simulink model "Simulink_30_09"  (R2020a)
settings: Solver=VariableStepAuto  StartTime=0.0  StopTime=75  RelTol=1e-3
values from neighbouring files (symbols this model uses):
  K_LQR = Ks(:,[1:2])    [Script_LQR.m]    (also in Workspace_21_09.mat = [0.405324117713 1.57304723801]; Workspace_23_09.mat = [0.405324117713 1.57304723801]; Workspace_30_09.mat = [7.00831546655 5.45122974139]; Workspace_30_09_1.mat = [0.406231829475 1.23772711101])
  K_REI = [Ks(:,1) Ks(:,2)]    [Retro_Alimentacion_Integral.m]    (also in Workspace_30_09.mat = [5.59001533188 7.18657171923]; Workspace_30_09_1.mat = [5.59001533188 7.18657171923])
  Kd_ms = 0.1649    [Workspace_30_09.mat]    (also in Workspace_30_09_1.mat)
  Ki_LQR = -Ks(:,[3])    [Script_LQR.m]    (also in Workspace_21_09.mat = 1; Workspace_23_09.mat = 1; Workspace_30_09.mat = 5.9160797831; Workspace_30_09_1.mat = 1.18321595662)
  Ki_ms = 0.6328    [Workspace_30_09.mat]    (also in Workspace_30_09_1.mat)
  Ki_REI = -Ks(:,3)    [Retro_Alimentacion_Integral.m]    (also in Workspace_30_09.mat = 10.5317472521; Workspace_30_09_1.mat = 10.5317472521)
  Kp_ms = -0.2794    [Workspace_30_09.mat]    (also in Workspace_30_09_1.mat)
libraries: cstblocks x6, simulink x3
settings Model: Creator=geral  LastModifiedBy=geral

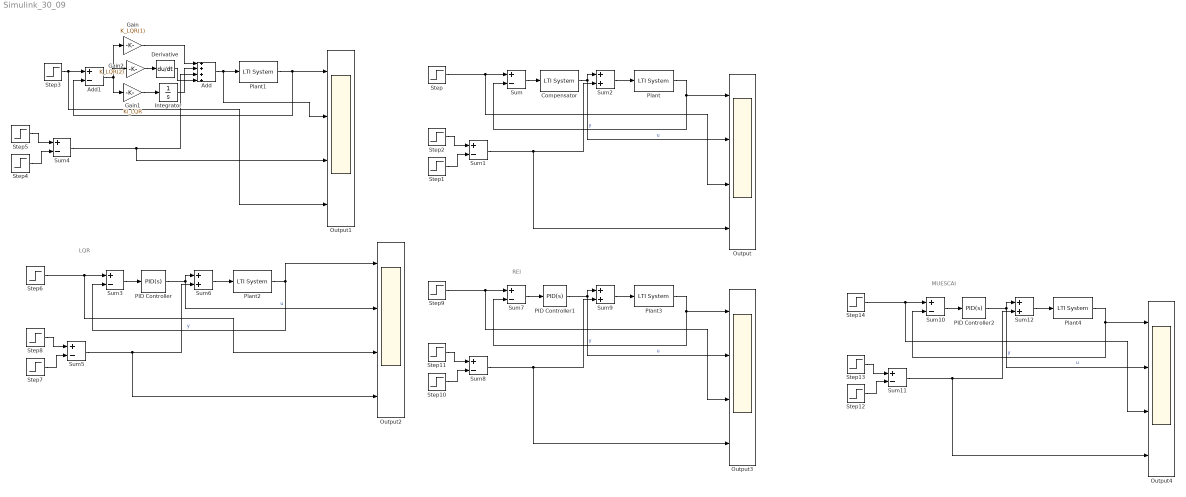
== system Simulink_30_09 ==
  note: REI
  note: LQR
  note: MUESCAI
  Add : Sum  Inputs=++++
  Add1 : Sum  Inputs=+-
  Compensator : cstblocks/LTI System  sys=C_IMC  IC=[]
  Derivative : Derivative
  Gain : Gain  Gain=K_LQR(1)
  Gain1 : Gain  Gain=Ki_LQR
  Gain2 : Gain  Gain=K_LQR(2)
  Integrator : Integrator
  Output{,1..4} (5 alike) : Scope  NumInputPorts=4
  PID Controller : simulink/Continuous/PID Controller  Controller=PID  Form=Parallel  TimeDomain=Continuous-time  UseExternalTs=off  SampleTime=-1  IntegratorMethod=Forward Euler  FilterMethod=Forward Euler  ControllerParametersSource=internal  P=K_LQR(1)  I=Ki_LQR  D=K_LQR(2)  UseFilter=on  N=15  TunerSelectOption=Transfer Function Based (PID Tuner App)  InitialConditionSource=internal  InitialConditionForIntegrator=0  InitialConditionForFilter=0  DifferentiatorICPrevScaledInput=0  ExternalReset=none  TrackingMode=off  Kt=1  LimitOutput=off  UpperSaturationLimit=inf  LowerSaturationLimit=-inf  LinearizeAsGain=on  AntiWindupMode=none  Kb=1  POutMin=[]  POutMax=[]  IOutMin=[]  IOutMax=[]  DOutMin=[]  DOutMax=[]  NOutMin=[]  NOutMax=[]  SumOutMin=[]  SumOutMax=[]  SaturationOutMin=[]  SaturationOutMax=[]  PParamMin=[]  PParamMax=[]  IParamMin=[]  IParamMax=[]  DParamMin=[]  DParamMax=[]  NParamMin=[]  NParamMax=[]  KbParamMin=[]  KbParamMax=[]  KtParamMin=[]  KtParamMax=[]  KbOutMin=[]  KbOutMax=[]  KtOutMin=[]  KtOutMax=[]  IntegratorOutMin=[]  IntegratorOutMax=[]  FilterOutMin=[]  FilterOutMax=[]  SumI1OutMin=[]  SumI1OutMax=[]  SumI2OutMin=[]  SumI2OutMax=[]  SumI3OutMin=[]  SumI3OutMax=[]  SumI4OutMin=[]  SumI4OutMax=[]  SumDOutMin=[]  SumDOutMax=[]  DifferentiatorOutMin=[]  DifferentiatorOutMax=[]  FilterDiffOutCoefMin=[]  FilterDiffOutCoefMax=[]  ReciprocalOutMin=[]  ReciprocalOutMax=[]  SumDenOutMin=[]  SumDenOutMax=[]  SumNumOutMin=[]  SumNumOutMax=[]  DivideOutMin=[]  DivideOutMax=[]  UdiffTsProdOutMin=[]  UdiffTsProdOutMax=[]  NTsProdOutMin=[]  NTsProdOutMax=[]  UintegralTsProdOutMin=[]  UintegralTsProdOutMax=[]  UngainTsProdOutMin=[]  UngainTsProdOutMax=[]  IntegratorContinuousStateAttributes=''  IntegratorStateMustResolveToSignalObject=off  IntegratorRTWStateStorageClass=Auto  FilterContinuousStateAttributes=''  FilterStateMustResolveToSignalObject=off  FilterRTWStateStorageClass=Auto  ParallelPVariant=InternalParameters  IdealPVariant=Disabled  IVariant=InternalParameters  DVariant=InternalParameters  IntegratorVariant=Continuous  SatVariant=Disabled  AWVariant=Passthrough  PCopyVariant=Disabled  TRVariant=Disabled  FdbkBlocksVariant=Forward  IdealPFdbkVariant=Disabled  SatFdbkVariant=Disabled  DerivativeFilterVariant=ContFilter  NVariant=InternalParameters  NCopyVariant=Disabled  FilterICVariant=InternalICsFilter  IntegratorICVariant=InternalICs  ExternalResetVariant=Disabled  TRSumVariant=Passthrough  SumFdbkVariant=Disabled  SumVariant=Sum_PID  TsampFilterVariant=InternalTs  TsampNgainVariant=Passthrough  TsampIntegralVariant=Passthrough
  PID Controller1 : simulink/Continuous/PID Controller  Controller=PID  Form=Parallel  TimeDomain=Continuous-time  UseExternalTs=off  SampleTime=-1  IntegratorMethod=Forward Euler  FilterMethod=Forward Euler  ControllerParametersSource=internal  P=K_REI(1)  I=Ki_REI  D=K_REI(2)  UseFilter=on  N=8.4  TunerSelectOption=Transfer Function Based (PID Tuner App)  InitialConditionSource=internal  InitialConditionForIntegrator=0  InitialConditionForFilter=0  DifferentiatorICPrevScaledInput=0  ExternalReset=none  TrackingMode=off  Kt=1  LimitOutput=off  UpperSaturationLimit=inf  LowerSaturationLimit=-inf  LinearizeAsGain=on  AntiWindupMode=none  Kb=1  POutMin=[]  POutMax=[]  IOutMin=[]  IOutMax=[]  DOutMin=[]  DOutMax=[]  NOutMin=[]  NOutMax=[]  SumOutMin=[]  SumOutMax=[]  SaturationOutMin=[]  SaturationOutMax=[]  PParamMin=[]  PParamMax=[]  IParamMin=[]  IParamMax=[]  DParamMin=[]  DParamMax=[]  NParamMin=[]  NParamMax=[]  KbParamMin=[]  KbParamMax=[]  KtParamMin=[]  KtParamMax=[]  KbOutMin=[]  KbOutMax=[]  KtOutMin=[]  KtOutMax=[]  IntegratorOutMin=[]  IntegratorOutMax=[]  FilterOutMin=[]  FilterOutMax=[]  SumI1OutMin=[]  SumI1OutMax=[]  SumI2OutMin=[]  SumI2OutMax=[]  SumI3OutMin=[]  SumI3OutMax=[]  SumI4OutMin=[]  SumI4OutMax=[]  SumDOutMin=[]  SumDOutMax=[]  DifferentiatorOutMin=[]  DifferentiatorOutMax=[]  FilterDiffOutCoefMin=[]  FilterDiffOutCoefMax=[]  ReciprocalOutMin=[]  ReciprocalOutMax=[]  SumDenOutMin=[]  SumDenOutMax=[]  SumNumOutMin=[]  SumNumOutMax=[]  DivideOutMin=[]  DivideOutMax=[]  UdiffTsProdOutMin=[]  UdiffTsProdOutMax=[]  NTsProdOutMin=[]  NTsProdOutMax=[]  UintegralTsProdOutMin=[]  UintegralTsProdOutMax=[]  UngainTsProdOutMin=[]  UngainTsProdOutMax=[]  IntegratorContinuousStateAttributes=''  IntegratorStateMustResolveToSignalObject=off  IntegratorRTWStateStorageClass=Auto  FilterContinuousStateAttributes=''  FilterStateMustResolveToSignalObject=off  FilterRTWStateStorageClass=Auto  ParallelPVariant=InternalParameters  IdealPVariant=Disabled  IVariant=InternalParameters  DVariant=InternalParameters  IntegratorVariant=Continuous  SatVariant=Disabled  AWVariant=Passthrough  PCopyVariant=Disabled  TRVariant=Disabled  FdbkBlocksVariant=Forward  IdealPFdbkVariant=Disabled  SatFdbkVariant=Disabled  DerivativeFilterVariant=ContFilter  NVariant=InternalParameters  NCopyVariant=Disabled  FilterICVariant=InternalICsFilter  IntegratorICVariant=InternalICs  ExternalResetVariant=Disabled  TRSumVariant=Passthrough  SumFdbkVariant=Disabled  SumVariant=Sum_PID  TsampFilterVariant=InternalTs  TsampNgainVariant=Passthrough  TsampIntegralVariant=Passthrough
  PID Controller2 : simulink/Continuous/PID Controller  Controller=PID  Form=Parallel  TimeDomain=Continuous-time  UseExternalTs=off  SampleTime=-1  IntegratorMethod=Forward Euler  FilterMethod=Forward Euler  ControllerParametersSource=internal  P=Kp_ms  I=Ki_ms  D=Kd_ms  UseFilter=on  N=30  TunerSelectOption=Transfer Function Based (PID Tuner App)  InitialConditionSource=internal  InitialConditionForIntegrator=0  InitialConditionForFilter=0  DifferentiatorICPrevScaledInput=0  ExternalReset=none  TrackingMode=off  Kt=1  LimitOutput=off  UpperSaturationLimit=inf  LowerSaturationLimit=-inf  LinearizeAsGain=on  AntiWindupMode=none  Kb=1  POutMin=[]  POutMax=[]  IOutMin=[]  IOutMax=[]  DOutMin=[]  DOutMax=[]  NOutMin=[]  NOutMax=[]  SumOutMin=[]  SumOutMax=[]  SaturationOutMin=[]  SaturationOutMax=[]  PParamMin=[]  PParamMax=[]  IParamMin=[]  IParamMax=[]  DParamMin=[]  DParamMax=[]  NParamMin=[]  NParamMax=[]  KbParamMin=[]  KbParamMax=[]  KtParamMin=[]  KtParamMax=[]  KbOutMin=[]  KbOutMax=[]  KtOutMin=[]  KtOutMax=[]  IntegratorOutMin=[]  IntegratorOutMax=[]  FilterOutMin=[]  FilterOutMax=[]  SumI1OutMin=[]  SumI1OutMax=[]  SumI2OutMin=[]  SumI2OutMax=[]  SumI3OutMin=[]  SumI3OutMax=[]  SumI4OutMin=[]  SumI4OutMax=[]  SumDOutMin=[]  SumDOutMax=[]  DifferentiatorOutMin=[]  DifferentiatorOutMax=[]  FilterDiffOutCoefMin=[]  FilterDiffOutCoefMax=[]  ReciprocalOutMin=[]  ReciprocalOutMax=[]  SumDenOutMin=[]  SumDenOutMax=[]  SumNumOutMin=[]  SumNumOutMax=[]  DivideOutMin=[]  DivideOutMax=[]  UdiffTsProdOutMin=[]  UdiffTsProdOutMax=[]  NTsProdOutMin=[]  NTsProdOutMax=[]  UintegralTsProdOutMin=[]  UintegralTsProdOutMax=[]  UngainTsProdOutMin=[]  UngainTsProdOutMax=[]  IntegratorContinuousStateAttributes=''  IntegratorStateMustResolveToSignalObject=off  IntegratorRTWStateStorageClass=Auto  FilterContinuousStateAttributes=''  FilterStateMustResolveToSignalObject=off  FilterRTWStateStorageClass=Auto  ParallelPVariant=InternalParameters  IdealPVariant=Disabled  IVariant=InternalParameters  DVariant=InternalParameters  IntegratorVariant=Continuous  SatVariant=Disabled  AWVariant=Passthrough  PCopyVariant=Disabled  TRVariant=Disabled  FdbkBlocksVariant=Forward  IdealPFdbkVariant=Disabled  SatFdbkVariant=Disabled  DerivativeFilterVariant=ContFilter  NVariant=InternalParameters  NCopyVariant=Disabled  FilterICVariant=InternalICsFilter  IntegratorICVariant=InternalICs  ExternalResetVariant=Disabled  TRSumVariant=Passthrough  SumFdbkVariant=Disabled  SumVariant=Sum_PID  TsampFilterVariant=InternalTs  TsampNgainVariant=Passthrough  TsampIntegralVariant=Passthrough
  Plant{,1..4} (5 alike) : cstblocks/LTI System  sys=tf10  IC=[]
  Step{,3,6,9,14} (5 alike) : Step  Time=0.1  After=0.7  SampleTime=0
  Step1 : Step  Time=25  After=0.1  SampleTime=0
  Step10 : Step  Time=40  After=0.1  SampleTime=0
  Step{4,8,11,13} (4 alike) : Step  Time=35  After=0.1  SampleTime=0
  Step12 : Step  Time=40  After=0.1  SampleTime=0
  Step2 : Step  Time=20  After=0.1  SampleTime=0
  Step5 : Step  Time=30  After=0.1  SampleTime=0
  Step7 : Step  Time=40  After=0.1  SampleTime=0
  Sum{,1,3..5,7..8,10..11} (9 alike) : Sum  Inputs=+-
  Sum{2,6,9,12} (4 alike) : Sum
  wires:
  Sum/1 -> Compensator/1
  Plant/1 -> Sum/2, Output/1  "y"
  Step/1 -> Output/3, Sum/1
  Step2/1 -> Sum1/1
  Step1/1 -> Sum1/2
  Sum2/1 -> Plant/1
  Compensator/1 -> Output/2, Sum2/1  "u"
  Sum1/1 -> Output/4, Sum2/2
  Step4/1 -> Sum4/2
  Step5/1 -> Sum4/1
  Plant1/1 -> Add1/2, Output1/1
  Gain1/1 -> Integrator/1
  Add/1 -> Output1/2, Plant1/1
  Integrator/1 -> Add/2
  Gain/1 -> Add/1
  Step3/1 -> Output1/4, Add1/1
  Add1/1 -> Gain1/1, Gain2/1, Gain/1
  Sum4/1 -> Output1/3, Add/3
  Gain2/1 -> Derivative/1
  Derivative/1 -> Add/4
  Step8/1 -> Sum5/1
  Sum6/1 -> Plant2/1
  Sum5/1 -> Output2/4, Sum6/2
  Plant2/1 -> Sum3/2, Output2/1  "y"
  PID Controller/1 -> Output2/2, Sum6/1  "u"
  Step6/1 -> Output2/3, Sum3/1
  Step7/1 -> Sum5/2
  Sum3/1 -> PID Controller/1
  PID Controller1/1 -> Output3/2, Sum9/1  "u"
  Sum7/1 -> PID Controller1/1
  Sum9/1 -> Plant3/1
  Step11/1 -> Sum8/1
  Step9/1 -> Output3/3, Sum7/1
  Plant3/1 -> Sum7/2, Output3/1  "y"
  Sum8/1 -> Output3/4, Sum9/2
  Step10/1 -> Sum8/2
  Sum11/1 -> Output4/4, Sum12/2
  Step12/1 -> Sum11/2
  Plant4/1 -> Sum10/2, Output4/1  "y"
  PID Controller2/1 -> Output4/2, Sum12/1  "u"
  Sum10/1 -> PID Controller2/1
  Step13/1 -> Sum11/1
  Step14/1 -> Output4/3, Sum10/1
  Sum12/1 -> Plant4/1
